simulink model "CACC_sim"  (R2019b)
settings: Solver=ode45  StartTime=0.0  StopTime=120  MaxStep=0.01  RelTol=1e-3
values from neighbouring files (symbols this model uses):
  a_des_max = 5    [HW2_main.m]    (also in main.m)
  a_des_min = -3    [HW2_main.m]    (also in main.m)
  d_0 = 8    [HW2_main.m]    (also in main.m)
  K_a = 0.2    [HW2_main.m]    (also in main.m)
  K_d_err = 0.2    [HW2_main.m]    (also in main.m)
  K_v = 0.5    [HW2_main.m]    (also in main.m)
  K_v_r = 1.5    [HW2_main.m]    (also in main.m = 3)
  t_h_tar = 1    [HW2_main.m]    (also in main.m)
  v1_0 = 30    [HW2_main.m]    (also in main.m)
  v2_0 = 25    [HW2_main.m]    (also in main.m)
  v3_0 = 28    [HW2_main.m]    (also in main.m)
  v4_0 = 0    [HW2_main.m]    (also in main.m)
  v_tar = 30    [HW2_main.m]    (also in main.m)
  x1_0 = 150    [HW2_main.m]    (also in main.m)
  x2_0 = 100    [HW2_main.m]    (also in main.m)
  x3_0 = 50    [HW2_main.m]    (also in main.m)
  x4_0 = 0    [HW2_main.m]    (also in main.m)
undefined symbols (not defined in the file or in its folder): sigbuilder_block
libraries: cstblocks x4
settings Model: Creator=user  LastModifiedBy=user

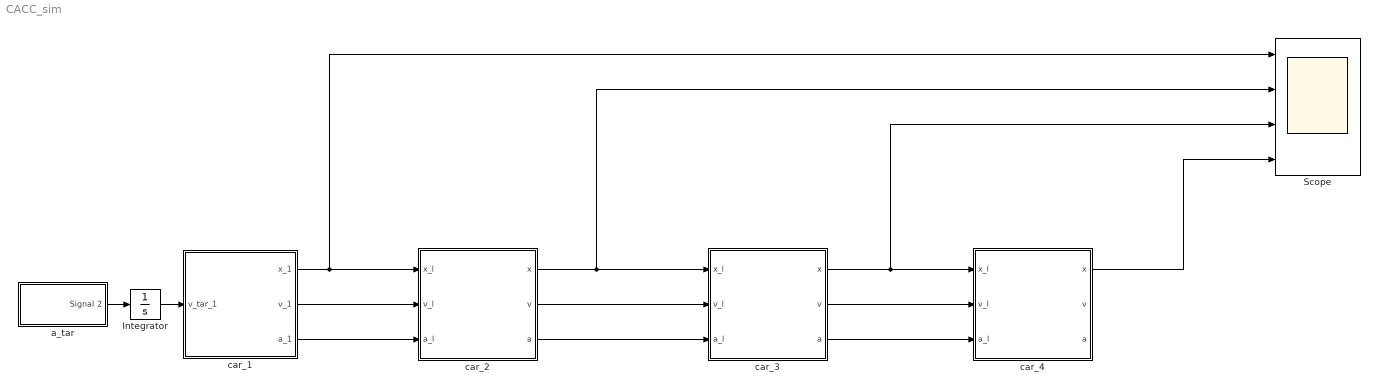
== system CACC_sim ==
  Integrator : Integrator
  Scope : Scope  NumInputPorts=4
  a_tar : Subsystem  Tag=STV Subsys  LoadFcn=sigbuilder_block('load');  StartFcn=sigbuilder_block('start');  StopFcn=sigbuilder_block('stop');  ClipboardFcn=sigbuilder_block('clipboard');  mask(Sigbuilder block){tuvar=[0:10]}
      mask help: Simulink:masks:SigbuilderBlock_MD
      mask init:
      | if ~strcmp(get_param(bdroot(gcbh),'SimulationStatus'),'stopped') tuvar = sigbuilder_block('maskInit'); end
      settings: CopyFcn=sigbuilder_block('copy');  DeleteFcn=sigbuilder_block('delete');  ModelCloseFcn=sigbuilder_block('modelClose');  PreSaveFcn=sigbuilder_block('preSave');  PauseFcn=sigbuilder_block('pause');  ContinueFcn=sigbuilder_block('continue');  NameChangeFcn=sigbuilder_block('namechange');  OpenFcn=sigbuilder_block('open',[287 48 550.5 362.5 ]);  CloseFcn=sigbuilder_block('close');
      mask Display: plot(0, 0, 100, 100,[2, 2, 32, 32, 2], [68, 8, 8, 68, 68],[32, 2], [38, 38], [32, 19, 2],[53, 60, 44], [32, 17, 17, 2],[16, 16, 31, 31]);txt = getActiveGroup(gcbh);text(2, 100, txt,'verticalAlignment', 'top');
  car_1 : Subsystem
  car_2 : Subsystem
  car_3 : Subsystem
  car_4 : Subsystem
  wires:
  a_tar/1(Signal 2) -> Integrator/1
  car_1/2(v_1) -> car_2/2(v_l)
  car_2/1(x) -> car_3/1(x_l), Scope/2
  car_2/2(v) -> car_3/2(v_l)
  car_1/1(x_1) -> car_2/1(x_l), Scope/1
  car_1/3(a_1) -> car_2/3(a_l)
  car_2/3(a) -> car_3/3(a_l)
  car_3/3(a) -> car_4/3(a_l)
  car_3/2(v) -> car_4/2(v_l)
  car_3/1(x) -> car_4/1(x_l), Scope/3
  car_4/1(x) -> Scope/4
  Integrator/1 -> car_1/1(v_tar_1)

== system CACC_sim/a_tar ==
  Demux : Demux  Tag=STV Demux  Outputs=1
  FromWs : FromWorkspace  Tag=STV FromWs  VariableName=tuvar  SampleTime=0
      SigBuilderData=|
      | common.afterFinalStr = 'Extrapolate'
      | common.sampleTime = 0
      | dataSet.timeRange = [0 120]
      | dataSet.name = 'Group 1'
      | sbobj.Groups.Name = 'Group 1'
      | sbobj.Groups.Signals.Name = 'Signal 2'
      | sbobj.Groups.Signals.XData = [0 10 10.5 13.5 14 40 40.5 43.5 44 60 70 70.5 73.5 74 100 100.5 103.5 104 120]
      | sbobj.Groups.Signals.YData = [0 0 -2 -2 0 0 2 2 0 0 0 -2 -2 0 0 2 2 0 0]
      | sbobj.Groups.TimeRange = [0 120]
  Signal 2 : Outport  Tag=STV Outport
  wires:
  FromWs/1 -> Demux/1
  Demux/1 -> Signal 2/1

== system CACC_sim/car_1 ==
  v_tar_1 : Inport
  vehicle 1 : Subsystem
  velocity_control : Subsystem
  x_1 : Outport
  v_1 : Outport  Port=2
  a_1 : Outport  Port=3
  wires:
  vehicle 1/3(v) -> v_1/1, velocity_control/2(v_h)
  velocity_control/1(a_des) -> vehicle 1/1(a_des)
  vehicle 1/2(a) -> a_1/1
  v_tar_1/1 -> velocity_control/1(v_tar)
  vehicle 1/1(x) -> x_1/1

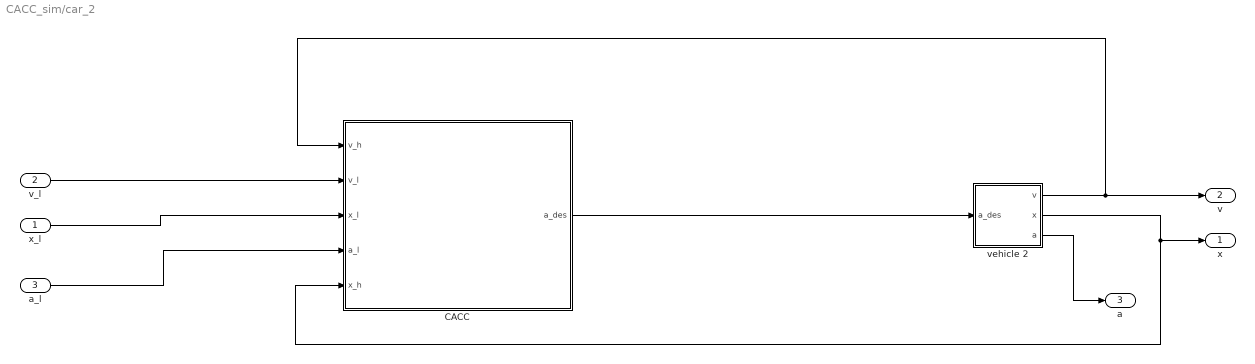
== system CACC_sim/car_2 ==
  x_l : Inport
  v_l : Inport  Port=2
  a_l : Inport  Port=3
  CACC : Subsystem
  vehicle 2 : Subsystem
  x : Outport
  v : Outport  Port=2
  a : Outport  Port=3
  wires:
  vehicle 2/1(v) -> v/1, CACC/1(v_h)
  v_l/1 -> CACC/2(v_l)
  x_l/1 -> CACC/3(x_l)
  CACC/1(a_des) -> vehicle 2/1(a_des)
  a_l/1 -> CACC/4(a_l)
  vehicle 2/3(a) -> a/1
  vehicle 2/2(x) -> CACC/5(x_h), x/1

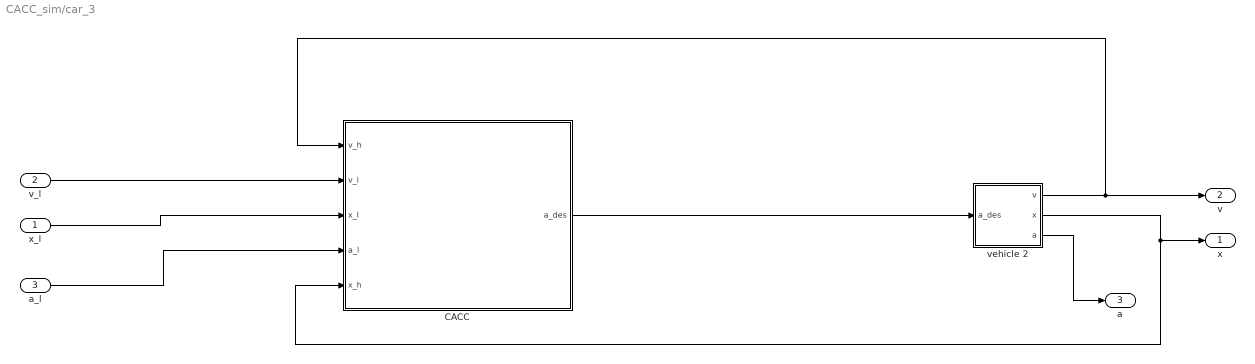
== system CACC_sim/car_3 ==
  x_l : Inport
  v_l : Inport  Port=2
  a_l : Inport  Port=3
  CACC : Subsystem
  vehicle 2 : Subsystem
  x : Outport
  v : Outport  Port=2
  a : Outport  Port=3
  wires:
  vehicle 2/1(v) -> v/1, CACC/1(v_h)
  v_l/1 -> CACC/2(v_l)
  x_l/1 -> CACC/3(x_l)
  CACC/1(a_des) -> vehicle 2/1(a_des)
  a_l/1 -> CACC/4(a_l)
  vehicle 2/3(a) -> a/1
  vehicle 2/2(x) -> CACC/5(x_h), x/1

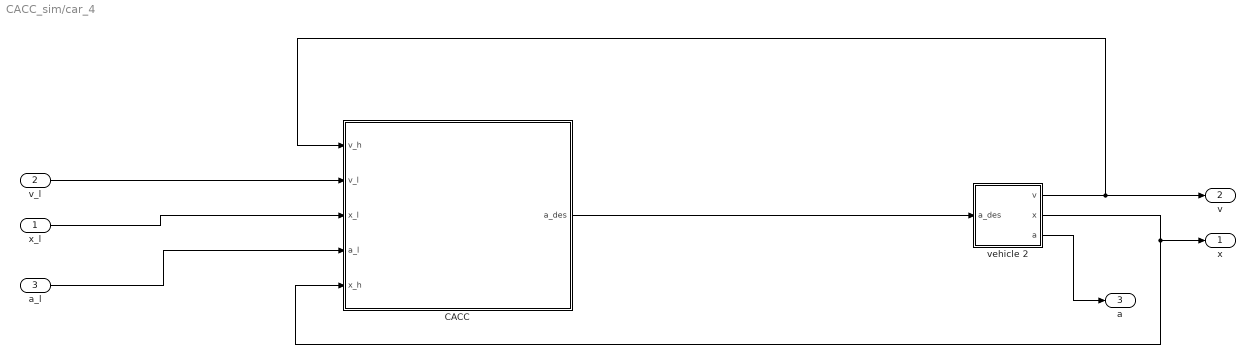
== system CACC_sim/car_4 ==
  x_l : Inport
  v_l : Inport  Port=2
  a_l : Inport  Port=3
  CACC : Subsystem
  vehicle 2 : Subsystem
  x : Outport
  v : Outport  Port=2
  a : Outport  Port=3
  wires:
  vehicle 2/1(v) -> v/1, CACC/1(v_h)
  v_l/1 -> CACC/2(v_l)
  x_l/1 -> CACC/3(x_l)
  CACC/1(a_des) -> vehicle 2/1(a_des)
  a_l/1 -> CACC/4(a_l)
  vehicle 2/3(a) -> a/1
  vehicle 2/2(x) -> CACC/5(x_h), x/1

== system CACC_sim/car_1/vehicle 1 ==
  a_des : Inport
  LTI System : cstblocks/LTI System  sys=G_a  IC=[]
  V : Integrator  InitialCondition=v1_0
  X : Integrator  InitialCondition=x1_0
  x : Outport
  a : Outport  Port=2
  v : Outport  Port=3
  wires:
  X/1 -> x/1
  LTI System/1 -> a/1, V/1
  V/1 -> v/1, X/1
  a_des/1 -> LTI System/1

== system CACC_sim/car_1/velocity_control ==
  v_tar : Inport
  v_h : Inport  Port=2
  Gain : Gain  Gain=K_v
  Saturation : Saturate  UpperLimit=a_des_max  LowerLimit=a_des_min
  Sum : Sum  Inputs=|+-
  a_des : Outport
  wires:
  Gain/1 -> Saturation/1
  Sum/1 -> Gain/1
  v_tar/1 -> Sum/1
  v_h/1 -> Sum/2
  Saturation/1 -> a_des/1

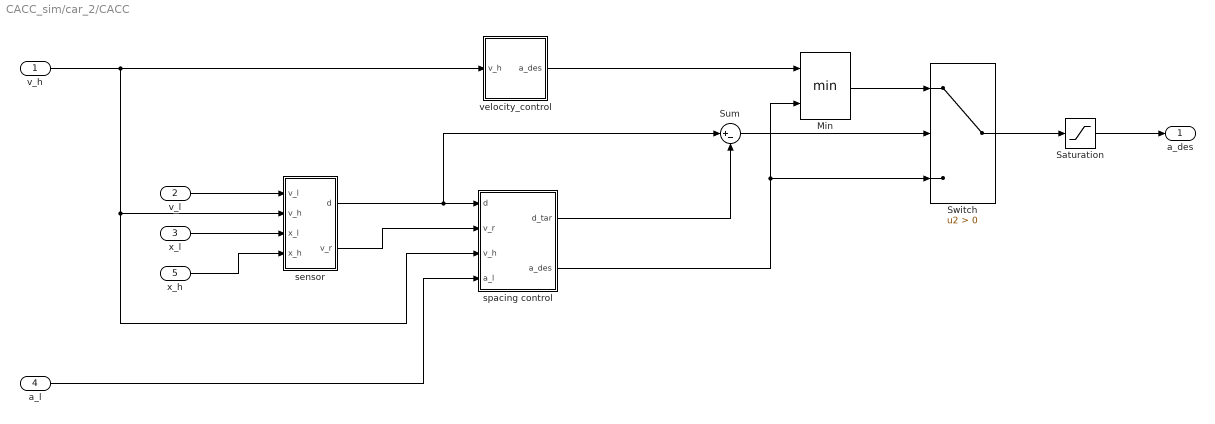
== system CACC_sim/car_2/CACC ==
  v_h : Inport
  v_l : Inport  Port=2
  x_l : Inport  Port=3
  a_l : Inport  Port=4
  x_h : Inport  Port=5
  Min : MinMax  Inputs=2
  Saturation : Saturate  UpperLimit=a_des_max  LowerLimit=a_des_min
  Sum : Sum  Inputs=|+-
  Switch : Switch  Criteria=u2 > Threshold
  sensor : Subsystem
  spacing control : Subsystem
  velocity_control : Subsystem
  a_des : Outport
  wires:
  sensor/2(v_r) -> spacing control/2(v_r)
  velocity_control/1(a_des) -> Min/1
  v_l/1 -> sensor/1(v_l)
  spacing control/1(d_tar) -> Sum/2
  sensor/1(d) -> Sum/1, spacing control/1(d)
  x_l/1 -> sensor/3(x_l)
  spacing control/2(a_des) -> Min/2, Switch/3
  v_h/1 -> velocity_control/1(v_h), sensor/2(v_h), spacing control/3(v_h)
  Min/1 -> Switch/1
  Sum/1 -> Switch/2
  Switch/1 -> Saturation/1
  x_h/1 -> sensor/4(x_h)
  a_l/1 -> spacing control/4(a_l)
  Saturation/1 -> a_des/1

== system CACC_sim/car_2/vehicle 2 ==
  a_des : Inport
  LTI System : cstblocks/LTI System  sys=G_a  IC=[]
  V : Integrator  InitialCondition=v2_0
  X : Integrator  InitialCondition=x2_0
  v : Outport
  x : Outport  Port=2
  a : Outport  Port=3
  wires:
  X/1 -> x/1
  LTI System/1 -> a/1, V/1
  V/1 -> v/1, X/1
  a_des/1 -> LTI System/1

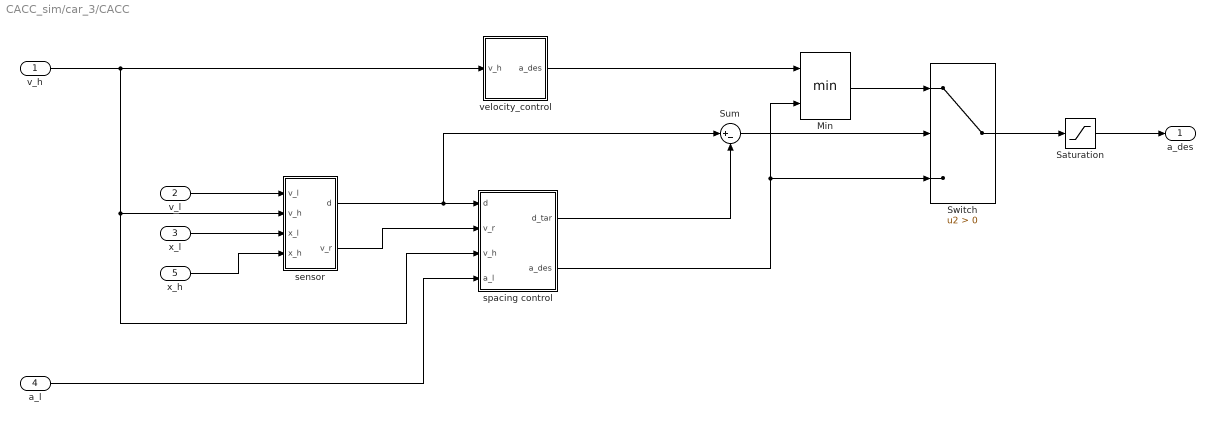
== system CACC_sim/car_3/CACC ==
  v_h : Inport
  v_l : Inport  Port=2
  x_l : Inport  Port=3
  a_l : Inport  Port=4
  x_h : Inport  Port=5
  Min : MinMax  Inputs=2
  Saturation : Saturate  UpperLimit=a_des_max  LowerLimit=a_des_min
  Sum : Sum  Inputs=|+-
  Switch : Switch  Criteria=u2 > Threshold
  sensor : Subsystem
  spacing control : Subsystem
  velocity_control : Subsystem
  a_des : Outport
  wires:
  sensor/2(v_r) -> spacing control/2(v_r)
  velocity_control/1(a_des) -> Min/1
  v_l/1 -> sensor/1(v_l)
  spacing control/1(d_tar) -> Sum/2
  sensor/1(d) -> Sum/1, spacing control/1(d)
  x_l/1 -> sensor/3(x_l)
  spacing control/2(a_des) -> Min/2, Switch/3
  v_h/1 -> velocity_control/1(v_h), sensor/2(v_h), spacing control/3(v_h)
  Min/1 -> Switch/1
  Sum/1 -> Switch/2
  Switch/1 -> Saturation/1
  x_h/1 -> sensor/4(x_h)
  a_l/1 -> spacing control/4(a_l)
  Saturation/1 -> a_des/1

== system CACC_sim/car_3/vehicle 2 ==
  a_des : Inport
  LTI System : cstblocks/LTI System  sys=G_a  IC=[]
  V : Integrator  InitialCondition=v3_0
  X : Integrator  InitialCondition=x3_0
  v : Outport
  x : Outport  Port=2
  a : Outport  Port=3
  wires:
  X/1 -> x/1
  LTI System/1 -> a/1, V/1
  V/1 -> v/1, X/1
  a_des/1 -> LTI System/1

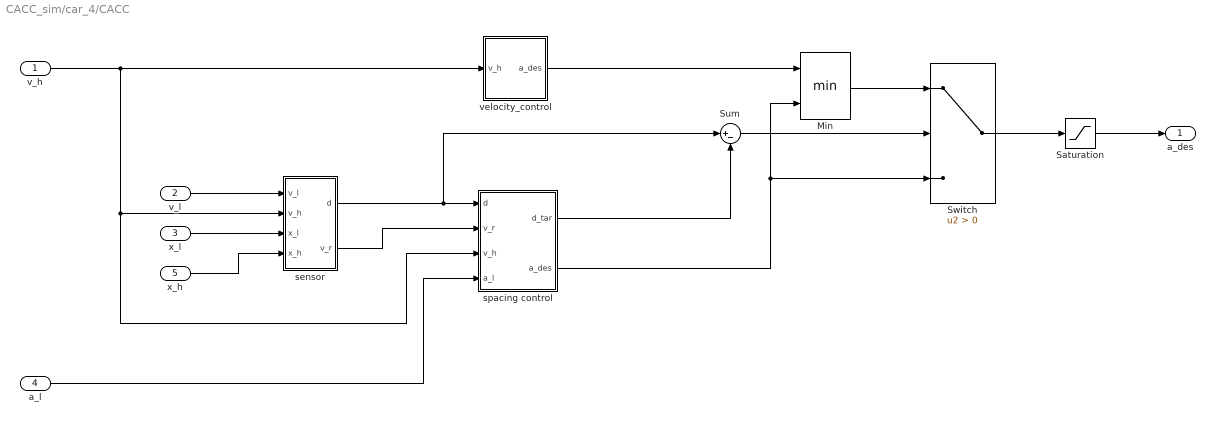
== system CACC_sim/car_4/CACC ==
  v_h : Inport
  v_l : Inport  Port=2
  x_l : Inport  Port=3
  a_l : Inport  Port=4
  x_h : Inport  Port=5
  Min : MinMax  Inputs=2
  Saturation : Saturate  UpperLimit=a_des_max  LowerLimit=a_des_min
  Sum : Sum  Inputs=|+-
  Switch : Switch  Criteria=u2 > Threshold
  sensor : Subsystem
  spacing control : Subsystem
  velocity_control : Subsystem
  a_des : Outport
  wires:
  sensor/2(v_r) -> spacing control/2(v_r)
  velocity_control/1(a_des) -> Min/1
  v_l/1 -> sensor/1(v_l)
  spacing control/1(d_tar) -> Sum/2
  sensor/1(d) -> Sum/1, spacing control/1(d)
  x_l/1 -> sensor/3(x_l)
  spacing control/2(a_des) -> Min/2, Switch/3
  v_h/1 -> velocity_control/1(v_h), sensor/2(v_h), spacing control/3(v_h)
  Min/1 -> Switch/1
  Sum/1 -> Switch/2
  Switch/1 -> Saturation/1
  x_h/1 -> sensor/4(x_h)
  a_l/1 -> spacing control/4(a_l)
  Saturation/1 -> a_des/1

== system CACC_sim/car_4/vehicle 2 ==
  a_des : Inport
  LTI System : cstblocks/LTI System  sys=G_a  IC=[]
  V : Integrator  InitialCondition=v4_0
  X : Integrator  InitialCondition=x4_0
  v : Outport
  x : Outport  Port=2
  a : Outport  Port=3
  wires:
  X/1 -> x/1
  LTI System/1 -> a/1, V/1
  V/1 -> v/1, X/1
  a_des/1 -> LTI System/1

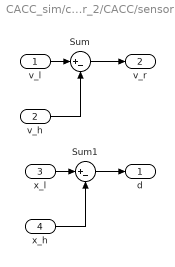
== system CACC_sim/car_2/CACC/sensor ==
  v_l : Inport
  v_h : Inport  Port=2
  x_l : Inport  Port=3
  x_h : Inport  Port=4
  Sum : Sum  Inputs=|+-
  Sum1 : Sum  Inputs=|+-
  d : Outport
  v_r : Outport  Port=2
  wires:
  Sum/1 -> v_r/1
  x_l/1 -> Sum1/1
  x_h/1 -> Sum1/2
  v_l/1 -> Sum/1
  v_h/1 -> Sum/2
  Sum1/1 -> d/1

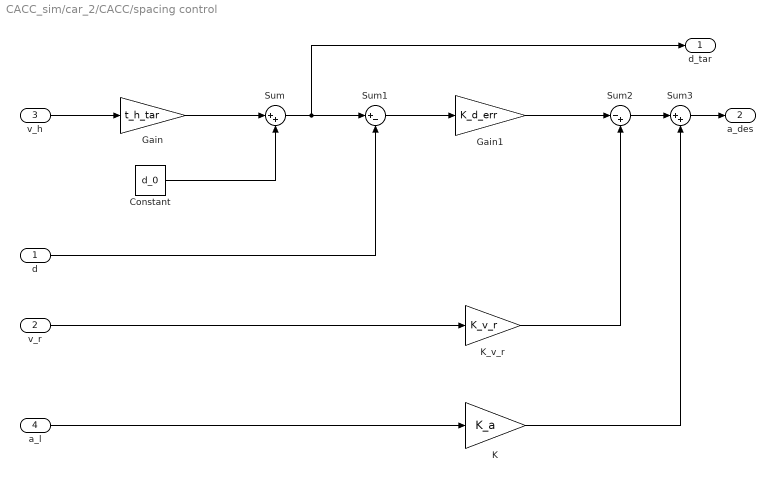
== system CACC_sim/car_2/CACC/spacing control ==
  d : Inport
  v_r : Inport  Port=2
  v_h : Inport  Port=3
  a_l : Inport  Port=4
  Constant : Constant  Value=d_0
  Gain : Gain  Gain=t_h_tar
  Gain1 : Gain  Gain=K_d_err
  K : Gain  Gain=K_a
  K_v_r : Gain  Gain=K_v_r
  Sum : Sum  Inputs=|++
  Sum1 : Sum  Inputs=|+-
  Sum2 : Sum  Inputs=|-+
  Sum3 : Sum  Inputs=|++
  d_tar : Outport
  a_des : Outport  Port=2
  wires:
  v_h/1 -> Gain/1
  Gain/1 -> Sum/1
  Constant/1 -> Sum/2
  Sum/1 -> d_tar/1, Sum1/1
  d/1 -> Sum1/2
  Sum1/1 -> Gain1/1
  v_r/1 -> K_v_r/1
  Gain1/1 -> Sum2/1
  K_v_r/1 -> Sum2/2
  a_l/1 -> K/1
  Sum2/1 -> Sum3/1
  K/1 -> Sum3/2
  Sum3/1 -> a_des/1

== system CACC_sim/car_2/CACC/velocity_control ==
  v_h : Inport
  Constant : Constant  Value=v_tar
  Gain : Gain  Gain=K_v
  Sum : Sum  Inputs=|+-
  a_des : Outport
  wires:
  v_h/1 -> Sum/2
  Constant/1 -> Sum/1
  Sum/1 -> Gain/1
  Gain/1 -> a_des/1

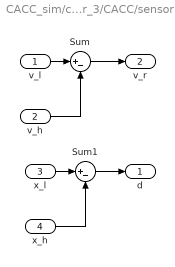
== system CACC_sim/car_3/CACC/sensor ==
  v_l : Inport
  v_h : Inport  Port=2
  x_l : Inport  Port=3
  x_h : Inport  Port=4
  Sum : Sum  Inputs=|+-
  Sum1 : Sum  Inputs=|+-
  d : Outport
  v_r : Outport  Port=2
  wires:
  Sum/1 -> v_r/1
  x_l/1 -> Sum1/1
  x_h/1 -> Sum1/2
  v_l/1 -> Sum/1
  v_h/1 -> Sum/2
  Sum1/1 -> d/1

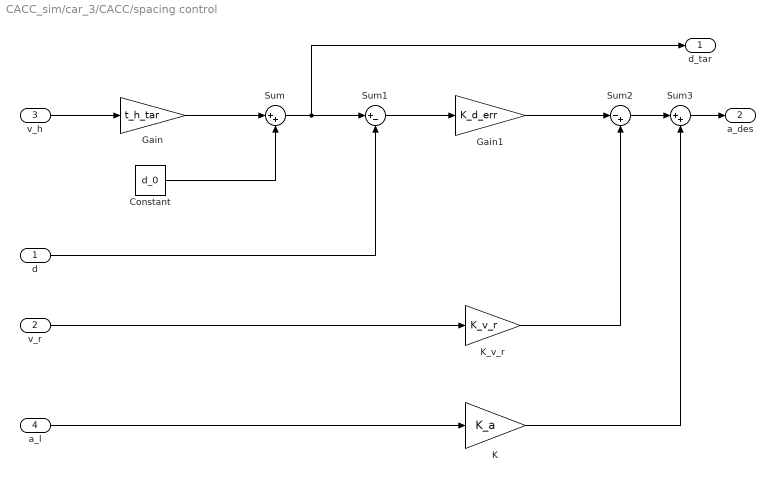
== system CACC_sim/car_3/CACC/spacing control ==
  d : Inport
  v_r : Inport  Port=2
  v_h : Inport  Port=3
  a_l : Inport  Port=4
  Constant : Constant  Value=d_0
  Gain : Gain  Gain=t_h_tar
  Gain1 : Gain  Gain=K_d_err
  K : Gain  Gain=K_a
  K_v_r : Gain  Gain=K_v_r
  Sum : Sum  Inputs=|++
  Sum1 : Sum  Inputs=|+-
  Sum2 : Sum  Inputs=|-+
  Sum3 : Sum  Inputs=|++
  d_tar : Outport
  a_des : Outport  Port=2
  wires:
  v_h/1 -> Gain/1
  Gain/1 -> Sum/1
  Constant/1 -> Sum/2
  Sum/1 -> d_tar/1, Sum1/1
  d/1 -> Sum1/2
  Sum1/1 -> Gain1/1
  v_r/1 -> K_v_r/1
  Gain1/1 -> Sum2/1
  K_v_r/1 -> Sum2/2
  a_l/1 -> K/1
  Sum2/1 -> Sum3/1
  K/1 -> Sum3/2
  Sum3/1 -> a_des/1

== system CACC_sim/car_3/CACC/velocity_control ==
  v_h : Inport
  Constant : Constant  Value=v_tar
  Gain : Gain  Gain=K_v
  Sum : Sum  Inputs=|+-
  a_des : Outport
  wires:
  v_h/1 -> Sum/2
  Constant/1 -> Sum/1
  Sum/1 -> Gain/1
  Gain/1 -> a_des/1

== system CACC_sim/car_4/CACC/sensor ==
  v_l : Inport
  v_h : Inport  Port=2
  x_l : Inport  Port=3
  x_h : Inport  Port=4
  Sum : Sum  Inputs=|+-
  Sum1 : Sum  Inputs=|+-
  d : Outport
  v_r : Outport  Port=2
  wires:
  Sum/1 -> v_r/1
  x_l/1 -> Sum1/1
  x_h/1 -> Sum1/2
  v_l/1 -> Sum/1
  v_h/1 -> Sum/2
  Sum1/1 -> d/1

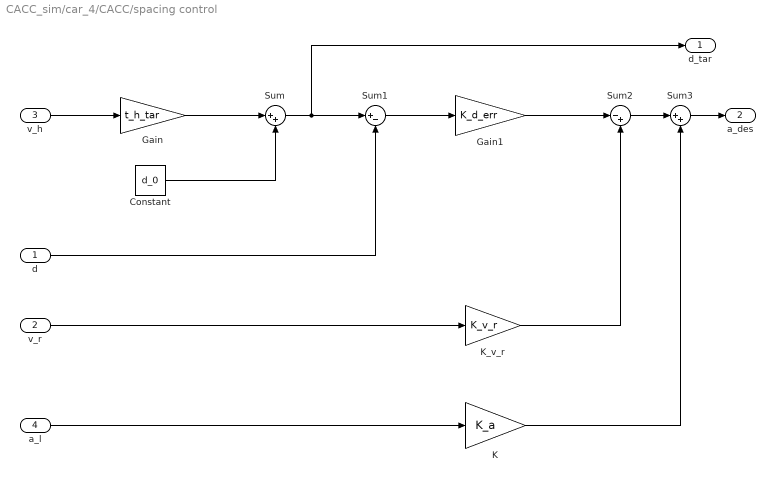
== system CACC_sim/car_4/CACC/spacing control ==
  d : Inport
  v_r : Inport  Port=2
  v_h : Inport  Port=3
  a_l : Inport  Port=4
  Constant : Constant  Value=d_0
  Gain : Gain  Gain=t_h_tar
  Gain1 : Gain  Gain=K_d_err
  K : Gain  Gain=K_a
  K_v_r : Gain  Gain=K_v_r
  Sum : Sum  Inputs=|++
  Sum1 : Sum  Inputs=|+-
  Sum2 : Sum  Inputs=|-+
  Sum3 : Sum  Inputs=|++
  d_tar : Outport
  a_des : Outport  Port=2
  wires:
  v_h/1 -> Gain/1
  Gain/1 -> Sum/1
  Constant/1 -> Sum/2
  Sum/1 -> d_tar/1, Sum1/1
  d/1 -> Sum1/2
  Sum1/1 -> Gain1/1
  v_r/1 -> K_v_r/1
  Gain1/1 -> Sum2/1
  K_v_r/1 -> Sum2/2
  a_l/1 -> K/1
  Sum2/1 -> Sum3/1
  K/1 -> Sum3/2
  Sum3/1 -> a_des/1

== system CACC_sim/car_4/CACC/velocity_control ==
  v_h : Inport
  Constant : Constant  Value=v_tar
  Gain : Gain  Gain=K_v
  Sum : Sum  Inputs=|+-
  a_des : Outport
  wires:
  v_h/1 -> Sum/2
  Constant/1 -> Sum/1
  Sum/1 -> Gain/1
  Gain/1 -> a_des/1
